simulink model "Lagr_Model_"  (R2022a)
settings: Solver=VariableStepAuto  StartTime=0.0  StopTime=100  RelTol=1e-3
values from neighbouring files (symbols this model uses):
  b1_damp = 0.5    [variable_for_simulink.m]
  b2_damp = 0.5    [variable_for_simulink.m]
  center1 = 0.216    [variable_for_simulink.m]
  center2 = 0.216    [variable_for_simulink.m]
  gravity = 9.8    [variable_for_simulink.m]
  inertia1 = 0.247    [variable_for_simulink.m]
  inertia2 = 0.177    [variable_for_simulink.m]
  length1 = 0.432    [variable_for_simulink.m]
  mass1 = 15.91    [variable_for_simulink.m]
  mass2 = 11.36    [variable_for_simulink.m]
settings Model: Creator=Steve  LastModifiedBy=Steve

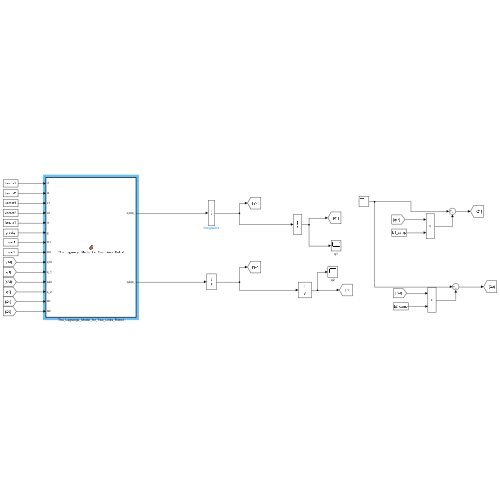
[thumbnail: Simulink's stored preview of the top-level diagram]
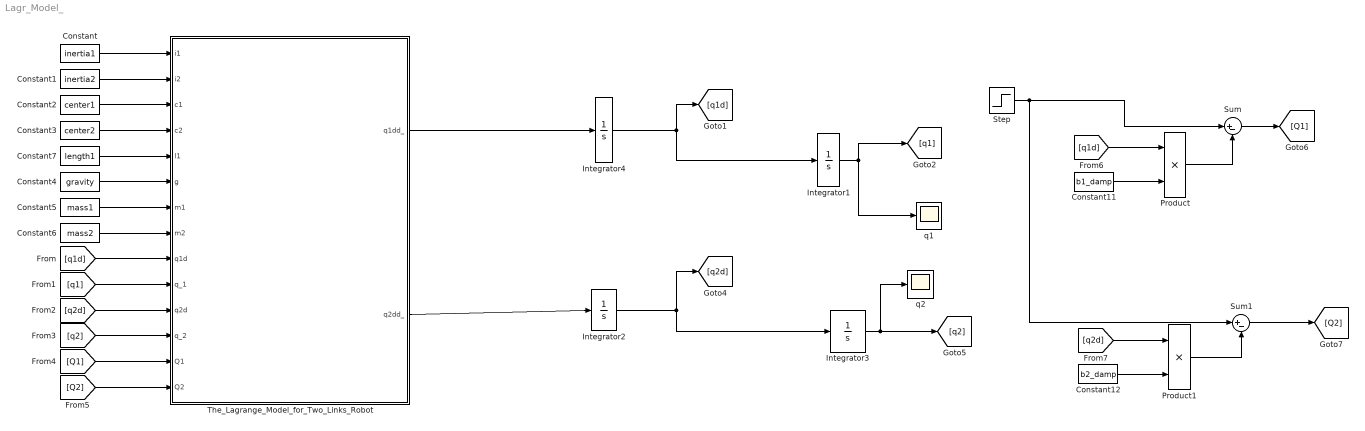
== system Lagr_Model_ ==
  Constant : Constant  Value=inertia1
  Constant1 : Constant  Value=inertia2
  Constant11 : Constant  Value=b1_damp
  Constant12 : Constant  Value=b2_damp
  Constant2 : Constant  Value=center1
  Constant3 : Constant  Value=center2
  Constant4 : Constant  Value=gravity
  Constant5 : Constant  Value=mass1
  Constant6 : Constant  Value=mass2
  Constant7 : Constant  Value=length1
  Integrator{1..4} (4 alike) : Integrator
  Product : Product
  Product1 : Product
  Step : Step  Before=1  After=0  SampleTime=0
  Sum : Sum  Inputs=|+-
  Sum1 : Sum  Inputs=|+-
  The_Lagrange_Model_for_Two_Links_Robot : MATLAB Function  TreatAsAtomicUnit=on
  q1 : Scope
  q2 : Scope
  wires:
  Constant4/1 -> The_Lagrange_Model_for_Two_Links_Robot/6(g)
  Constant1/1 -> The_Lagrange_Model_for_Two_Links_Robot/2(i2)
  Constant3/1 -> The_Lagrange_Model_for_Two_Links_Robot/4(c2)
  Constant/1 -> The_Lagrange_Model_for_Two_Links_Robot/1(i1)
  Constant2/1 -> The_Lagrange_Model_for_Two_Links_Robot/3(c1)
  Constant7/1 -> The_Lagrange_Model_for_Two_Links_Robot/5(l1)
  Constant5/1 -> The_Lagrange_Model_for_Two_Links_Robot/7(m1)
  Constant6/1 -> The_Lagrange_Model_for_Two_Links_Robot/8(m2)
  [q1d] -> The_Lagrange_Model_for_Two_Links_Robot/9(q1d)
  [q1] -> The_Lagrange_Model_for_Two_Links_Robot/10(q_1)
  [q2d] -> The_Lagrange_Model_for_Two_Links_Robot/11(q2d)
  [q2] -> The_Lagrange_Model_for_Two_Links_Robot/12(q_2)
  [Q1] -> The_Lagrange_Model_for_Two_Links_Robot/13(Q1)
  [Q2] -> The_Lagrange_Model_for_Two_Links_Robot/14(Q2)
  Integrator4/1 -> Integrator1/1, [q1d]
  Step/1 -> Sum/1, Sum1/1
  Sum/1 -> [Q1]
  [q2d] -> Product1/1
  Integrator2/1 -> Integrator3/1, [q2d]
  Constant12/1 -> Product1/2
  Integrator1/1 -> [q1], q1/1
  Integrator3/1 -> q2/1, [q2]
  Product/1 -> Sum/2
  [q1d] -> Product/1
  Constant11/1 -> Product/2
  Product1/1 -> Sum1/2
  Sum1/1 -> [Q2]
  The_Lagrange_Model_for_Two_Links_Robot/1(q1dd_) -> Integrator4/1
  The_Lagrange_Model_for_Two_Links_Robot/2(q2dd_) -> Integrator2/1

== matlab function Lagr_Model_/The_Lagrange_Model_for_Two_Links_Robot ==
  data: i1 input; q1dd_ output; i2 input; c1 input; c2 input; l1 input; g input; m1 input; m2 input; q1d input; q_1 input; q2d input; q_2 input; Q1 input; Q2 input; q2dd_ output
function [q1dd_,q2dd_] = The_Lagrange_Model_for_Two_Links_Robot(i1,i2,c1,c2,l1,g,m1,m2,q1d,q_1,q2d,q_2,Q1,Q2)
%#codegen

%    This function was generated by the Symbolic Math Toolbox version 9.1.
%    30-Nov-2022 10:42:33

et1 = 1.0./(i1.*i2+i2.*l1.^2.*m2+c2.^2.*l1.^2.*m2.^2+c1.^2.*i2.*m1+c2.^2.*i1.*m2+c1.^2.*c2.^2.*m1.*m2-c2.^2.*l1.^2.*m2.^2.*cos(q_2).^2);
et2 = Q1.*i2-Q2.*i2+Q1.*c2.^2.*m2-Q2.*c2.^2.*m2+c2.^3.*l1.*m2.^2.*q1d.^2.*sin(q_2)+c2.^3.*l1.*m2.^2.*q2d.^2.*sin(q_2)-c2.^2.*g.*l1.*m2.^2.*cos(q_1)-Q2.*c2.*l1.*m2.*cos(q_2)-c1.*g.*i2.*m1.*cos(q_1)-g.*i2.*l1.*m2.*cos(q_1)+c2.^3.*l1.*m2.^2.*q1d.*q2d.*sin(q_2).*2.0+c2.^2.*g.*l1.*m2.^2.*cos(q_1+q_2).*cos(q_2)+c2.^2.*l1.^2.*m2.^2.*q1d.^2.*cos(q_2).*sin(q_2)-c1.*c2.^2.*g.*m1.*m2.*cos(q_1)+c2.*i2.*l1.*m2.*q1d.^2.*sin(q_2)+c2.*i2.*l1.*m2.*q2d.^2.*sin(q_2)+c2.*i2.*l1.*m2.*q1d.*q2d.*sin(q_2).*2.0;
q1dd_ = et1.*et2;
if nargout > 1
    et3 = Q1.*i2-Q2.*i1-Q2.*i2-Q2.*c1.^2.*m1+Q1.*c2.^2.*m2-Q2.*c2.^2.*m2-Q2.*l1.^2.*m2+c2.*l1.^3.*m2.^2.*q1d.^2.*sin(q_2)+c2.^3.*l1.*m2.^2.*q1d.^2.*sin(q_2)+c2.^3.*l1.*m2.^2.*q2d.^2.*sin(q_2)+c2.*g.*l1.^2.*m2.^2.*cos(q_1+q_2)-c2.^2.*g.*l1.*m2.^2.*cos(q_1)+c2.*g.*i1.*m2.*cos(q_1+q_2)+Q1.*c2.*l1.*m2.*cos(q_2)-Q2.*c2.*l1.*m2.*cos(q_2).*2.0-c1.*g.*i2.*m1.*cos(q_1)-g.*i2.*l1.*m2.*cos(q_1)+c2.^3.*l1.*m2.^2.*q1d.*q2d.*sin(q_2).*2.0+c2.^2.*g.*l1.*m2.^2.*cos(q_1+q_2).*cos(q_2)+c2.^2.*l1.^2.*m2.^2.*q1d.^2.*cos(q_2).*sin(q_2).*2.0;
    et4 = c2.^2.*l1.^2.*m2.^2.*q2d.^2.*cos(q_2).*sin(q_2)-c2.*g.*l1.^2.*m2.^2.*cos(q_1).*cos(q_2)+c1.^2.*c2.*g.*m1.*m2.*cos(q_1+q_2)-c1.*c2.^2.*g.*m1.*m2.*cos(q_1)+c2.*i1.*l1.*m2.*q1d.^2.*sin(q_2)+c2.*i2.*l1.*m2.*q1d.^2.*sin(q_2)+c2.*i2.*l1.*m2.*q2d.^2.*sin(q_2)+c2.^2.*l1.^2.*m2.^2.*q1d.*q2d.*cos(q_2).*sin(q_2).*2.0+c1.^2.*c2.*l1.*m1.*m2.*q1d.^2.*sin(q_2)+c2.*i2.*l1.*m2.*q1d.*q2d.*sin(q_2).*2.0-c1.*c2.*g.*l1.*m1.*m2.*cos(q_1).*cos(q_2);
    q2dd_ = -(et3+et4)./(i1.*i2+i2.*l1.^2.*m2+c2.^2.*l1.^2.*m2.^2+c1.^2.*i2.*m1+c2.^2.*i1.*m2+c1.^2.*c2.^2.*m1.*m2-c2.^2.*l1.^2.*m2.^2.*cos(q_2).^2);
end
